simulink model "SS_Fire"  (R2019b)
settings: Solver=VariableStepAuto  StartTime=0.0  StopTime=10.0  RelTol=1e-3
settings Model: Creator=toons  LastModifiedBy=toons

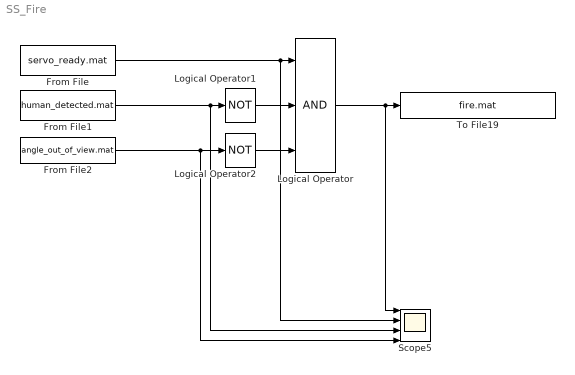
== system SS_Fire ==
  From File : FromFile  FileName=servo_ready.mat  SampleTime=0
  From File1 : FromFile  FileName=human_detected.mat  SampleTime=0
  From File2 : FromFile  FileName=angle_out_of_view.mat  SampleTime=0
  Logical Operator : Logic  Inputs=3  AllPortsSameDT=off  OutDataTypeStr=boolean
  Logical Operator1 : Logic  Operator=NOT  Inputs=3  AllPortsSameDT=off  OutDataTypeStr=boolean
  Logical Operator2 : Logic  Operator=NOT  Inputs=3  AllPortsSameDT=off  OutDataTypeStr=boolean
  Scope5 : Scope  NumInputPorts=4
  To File19 : ToFile  Filename=fire.mat  SaveFormat=Timeseries
  wires:
  Logical Operator/1 -> Scope5/1, To File19/1
  Logical Operator2/1 -> Logical Operator/3
  Logical Operator1/1 -> Logical Operator/2
  From File1/1 -> Scope5/3, Logical Operator1/1
  From File2/1 -> Logical Operator2/1, Scope5/4
  From File/1 -> Scope5/2, Logical Operator/1
